simulink model "KalmanAndOnBoardSensors"  (R2015a)
settings: Solver=ode45  StartTime=0.0  StopTime=10.0  RelTol=1e-3
undefined symbols (not defined in the file or in its folder): g, tc
settings Model: Creator=Mattia  LastModifiedBy=Mattia

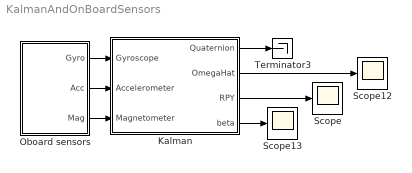
== system KalmanAndOnBoardSensors ==
  Kalman : Subsystem
  Oboard sensors : Subsystem
  Scope : Scope
      settings: SaveName=ScopeData8
  Scope12 : Scope
      settings: SaveName=ScopeData19
  Scope13 : Scope
      settings: SaveName=ScopeData23
  Terminator3 : Terminator
  wires:
  Kalman/1(Quaternion) -> Terminator3/1
  Kalman/2(OmegaHat) -> Scope12/1
  Kalman/3(RPY) -> Scope/1
  Kalman/4(beta) -> Scope13/1
  Oboard sensors/1(Gyro) -> Kalman/1(Gyroscope)
  Oboard sensors/2(Acc) -> Kalman/2(Accelerometer)
  Oboard sensors/3(Mag) -> Kalman/3("Magnetometer ")

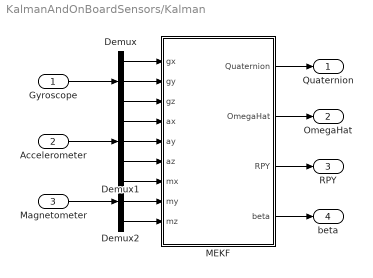
== system KalmanAndOnBoardSensors/Kalman ==
  Gyroscope : Inport
  Accelerometer : Inport  Port=2
  "Magnetometer " : Inport  Port=3
  Demux : Demux  Outputs=3
  Demux1 : Demux  Outputs=3
  Demux2 : Demux  Outputs=3
  MEKF : Subsystem
  Quaternion : Outport
  OmegaHat : Outport  Port=2
  RPY : Outport  Port=3
  beta : Outport  Port=4
  wires:
  Demux1/1 -> MEKF/4(ax)
  Demux1/2 -> MEKF/5(ay)
  Gyroscope/1 -> Demux/1
  Demux1/3 -> MEKF/6(az)
  Demux/3 -> MEKF/3(gz)
  Demux/2 -> MEKF/2(gy)
  Accelerometer/1 -> Demux1/1
  MEKF/2(OmegaHat) -> OmegaHat/1
  MEKF/1(Quaternion) -> Quaternion/1
  MEKF/3(RPY) -> RPY/1
  Demux2/1 -> MEKF/7(mx)
  "Magnetometer "/1 -> Demux2/1
  Demux2/2 -> MEKF/8(my)
  Demux2/3 -> MEKF/9(mz)
  Demux/1 -> MEKF/1(gx)
  MEKF/4("beta ") -> beta/1

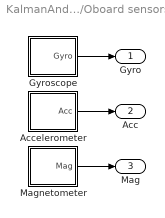
== system KalmanAndOnBoardSensors/Oboard sensors ==
  "Accelerometer " : Subsystem
  "Gyroscope " : Subsystem
  Magnetometer : Subsystem
  Gyro : Outport
  Acc : Outport  Port=2
  Mag : Outport  Port=3
  wires:
  "Gyroscope "/1(Gyro) -> Gyro/1
  "Accelerometer "/1(Acc) -> Acc/1
  Magnetometer/1(Mag) -> Mag/1

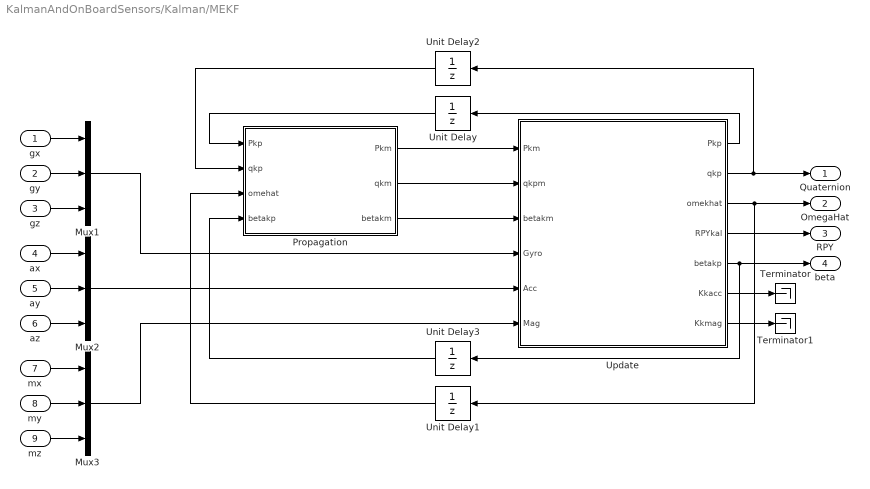
== system KalmanAndOnBoardSensors/Kalman/MEKF ==
  gx : Inport
  gy : Inport  Port=2
  gz : Inport  Port=3
  ax : Inport  Port=4
  ay : Inport  Port=5
  az : Inport  Port=6
  mx : Inport  Port=7
  my : Inport  Port=8
  mz : Inport  Port=9
  Mux1 : Mux  Inputs=3
  Mux2 : Mux  Inputs=3
  Mux3 : Mux  Inputs=3
  "Propagation " : MATLAB Function  TreatAsAtomicUnit=on
  Terminator : Terminator
  Terminator1 : Terminator
  Unit Delay : UnitDelay  InitialCondition=(1e-6)*eye(6)  SampleTime=-1
  Unit Delay1 : UnitDelay  InitialCondition=0.0000001*ones(3,1)  SampleTime=-1
  Unit Delay2 : UnitDelay  InitialCondition=[0 0 0 1]'  SampleTime=-1
  Unit Delay3 : UnitDelay  InitialCondition=0.0000001*ones(3,1)  SampleTime=-1
  Update : MATLAB Function  TreatAsAtomicUnit=on
  Quaternion : Outport
  OmegaHat : Outport  Port=2
  RPY : Outport  Port=3
  "beta " : Outport  Port=4
  wires:
  Update/1(Pkp) -> Unit Delay/1
  Update/3(omekhat) -> Unit Delay1/1, OmegaHat/1
  Unit Delay1/1 -> "Propagation "/3(omehat)
  Unit Delay/1 -> "Propagation "/1(Pkp)
  "Propagation "/1(Pkm) -> Update/1(Pkm)
  gx/1 -> Mux1/1
  gy/1 -> Mux1/2
  ax/1 -> Mux2/1
  mx/1 -> Mux3/1
  az/1 -> Mux2/3
  Update/2(qkp) -> Quaternion/1, Unit Delay2/1
  Update/5(betakp) -> Unit Delay3/1, "beta "/1
  gz/1 -> Mux1/3
  ay/1 -> Mux2/2
  Unit Delay2/1 -> "Propagation "/2(qkp)
  "Propagation "/2(qkm) -> Update/2(qkpm)
  mz/1 -> Mux3/3
  my/1 -> Mux3/2
  Mux1/1 -> Update/4(Gyro)
  Mux2/1 -> Update/5(Acc)
  Mux3/1 -> Update/6(Mag)
  Unit Delay3/1 -> "Propagation "/4(betakp)
  Update/4(RPYkal) -> RPY/1
  "Propagation "/3(betakm) -> Update/3(betakm)
  Update/6(Kkacc) -> Terminator/1
  Update/7(Kkmag) -> Terminator1/1

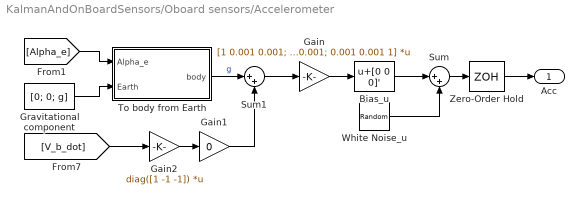
== system KalmanAndOnBoardSensors/Oboard sensors/Accelerometer  ==
  Bias_u : Bias  Bias=[0 0 0]'
  Gain : Gain  Gain=[1 0.001 0.001; 0.001 1 0.001; 0.001 0.001 1]  Multiplication=Matrix(K*u)
  Gain1 : Gain  Gain=0
  Gain2 : Gain  Gain=diag([1 -1 -1])  Multiplication=Matrix(K*u)
  Gravitational component : Constant  Value=[0; 0; g]
  Sum : Sum  Inputs=|++
  Sum1 : Sum  Inputs=|++
  To body from Earth : MATLAB Function  TreatAsAtomicUnit=on
  White Noise_u : RandomNumber  DisableCoverage=on  Variance=0*(0.02)^2  SampleTime=tc
  Zero-Order Hold : ZeroOrderHold  SampleTime=tc
  Acc : Outport
  wires:
  Gain/1 -> Bias_u/1
  Sum1/1 -> Gain/1
  Sum/1 -> Zero-Order Hold/1
  White Noise_u/1 -> Sum/2
  Zero-Order Hold/1 -> Acc/1
  Bias_u/1 -> Sum/1
  Gravitational component/1 -> To body from Earth/2(Earth)
  [Alpha_e] -> To body from Earth/1(Alpha_e)
  To body from Earth/1(body) -> Sum1/1  "g"
  Gain1/1 -> Sum1/2
  [V_b_dot] -> Gain2/1
  Gain2/1 -> Gain1/1

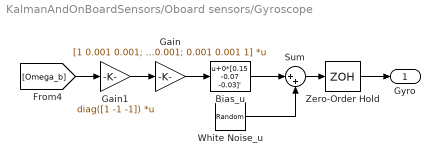
== system KalmanAndOnBoardSensors/Oboard sensors/Gyroscope  ==
  Bias_u : Bias  Bias=0*[0.15 -0.07 -0.03]'
  Gain : Gain  Gain=[1 0.001 0.001; 0.001 1 0.001; 0.001 0.001 1]  Multiplication=Matrix(K*u)
  Gain1 : Gain  Gain=diag([1 -1 -1])  Multiplication=Matrix(K*u)
  Sum : Sum  Inputs=|++
  White Noise_u : RandomNumber  DisableCoverage=on  Variance=0*(0.02)^2  SampleTime=tc
  Zero-Order Hold : ZeroOrderHold  SampleTime=tc
  Gyro : Outport
  wires:
  Bias_u/1 -> Sum/1
  Zero-Order Hold/1 -> Gyro/1
  White Noise_u/1 -> Sum/2
  Sum/1 -> Zero-Order Hold/1
  [Omega_b] -> Gain1/1
  Gain/1 -> Bias_u/1
  Gain1/1 -> Gain/1

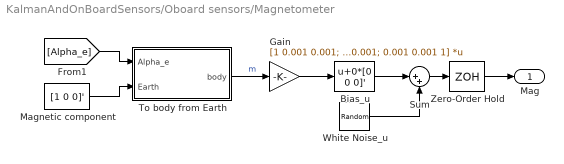
== system KalmanAndOnBoardSensors/Oboard sensors/Magnetometer ==
  Bias_u : Bias  Bias=0*[0 0 0]'
  Gain : Gain  Gain=[1 0.001 0.001; 0.001 1 0.001; 0.001 0.001 1]  Multiplication=Matrix(K*u)
  Magnetic component : Constant  Value=[1 0 0]'
  Sum : Sum  Inputs=|++
  To body from Earth : MATLAB Function  TreatAsAtomicUnit=on
  White Noise_u : RandomNumber  DisableCoverage=on  Variance=0*(0.02)^2  SampleTime=tc
  Zero-Order Hold : ZeroOrderHold  SampleTime=tc
  Mag : Outport
  wires:
  To body from Earth/1(body) -> Gain/1  "m"
  [Alpha_e] -> To body from Earth/1(Alpha_e)
  Magnetic component/1 -> To body from Earth/2(Earth)
  Bias_u/1 -> Sum/1
  Zero-Order Hold/1 -> Mag/1
  White Noise_u/1 -> Sum/2
  Sum/1 -> Zero-Order Hold/1
  Gain/1 -> Bias_u/1

== matlab function KalmanAndOnBoardSensors/Oboard sensors/Accelerometer /To body from Earth ==
  data: Alpha_e input; Earth input; body output
 function body = Tbe(Alpha_e, Earth)
%#codegen
phi = Alpha_e(1);
theta = Alpha_e(2);
psi = Alpha_e(3);

Sphi = sin(phi);
Cphi = cos(phi);
Stheta = sin(theta);
Ctheta = cos(theta);
Spsi = sin(psi);
Cpsi = cos(psi);

TBE = [        Ctheta*Cpsi               Ctheta*Spsi          -Stheta    ;
       Sphi*Stheta*Cpsi-Cphi*Spsi Sphi*Stheta*Spsi+Cphi*Cpsi Sphi*Ctheta ;
       Cphi*Stheta*Cpsi+Sphi*Spsi Cphi*Stheta*Spsi-Sphi*Cpsi Cphi*Ctheta];

body = TBE* Earth;

== matlab function KalmanAndOnBoardSensors/Oboard sensors/Magnetometer/To body from Earth ==
  data: Alpha_e input; Earth input; body output
 function body = Tbe(Alpha_e, Earth)
%#codegen
phi = Alpha_e(1);
theta = Alpha_e(2);
psi = Alpha_e(3);

Sphi = sin(phi);
Cphi = cos(phi);
Stheta = sin(theta);
Ctheta = cos(theta);
Spsi = sin(psi);
Cpsi = cos(psi);

TBE = [        Ctheta*Cpsi               Ctheta*Spsi          -Stheta    ;
       Sphi*Stheta*Cpsi-Cphi*Spsi Sphi*Stheta*Spsi+Cphi*Cpsi Sphi*Ctheta ;
       Cphi*Stheta*Cpsi+Sphi*Spsi Cphi*Stheta*Spsi-Sphi*Cpsi Cphi*Ctheta];

body = TBE* Earth;

== matlab function KalmanAndOnBoardSensors/Kalman/MEKF/Propagation  ==
  data Pkp settings: description=Control signal at the previous step.
  data qkp settings: description=Covariance estimate at the previous step.
  data Pkm settings: description=A-priori covariance estimate.
  data qkm settings: description=A-priori state estimate.
  data: Pkp input; qkp input; Pkm output; qkm output; omehat input; betakp input; betakm output
%% EKF - Propagation      %
% Author: Mattia Giurato  %
% Last review: 2016/03/15 %
%%%%%%%%%%%%%%%%%%%%%%%%%%%
function [Pkm,qkm,betakm] = Propagation(Pkp,qkp,omehat,betakp)
%% Usefull values
sigma_u = diag([0.13807 0.11053 0.063833/10])/100;
sigma_v = diag([0.00001 0.00001 0.05]);
dt = 0.01;

%% Quaternion propagation
omex = [     0      -omehat(3)  omehat(2) ;
         omehat(3)      0      -omehat(1) ;
        -omehat(2)  omehat(1)      0     ];
Omega = [  -omex   omehat ;
         -omehat'     0  ];
qt = (eye(4) + .5*Omega*dt)*qkp;
qkm = qt / sqrt(qt(1)^2+qt(2)^2+qt(3)^2+qt(4)^2);

%% Bias propagation
betakm = betakp;

%% Covariance equation propagation
omekhatx = [     0      -omehat(3)  omehat(2) ;
             omehat(3)     0       -omehat(1) ;
            -omehat(2)  omehat(1)      0     ];
nomehat = sqrt(omehat(1)^2+omehat(2)^2+omehat(3)^2);
Phi1 = eye(3) - omekhatx*sin(nomehat*dt)/nomehat + omekhatx*omekhatx*(1 - cos(nomehat*dt))/(nomehat^2);
Phi2 = omekhatx*(1 - cos(nomehat*dt))/(nomehat^2) - eye(3)*dt - omekhatx*omekhatx*(nomehat*dt - sin(nomehat*dt))/(nomehat^3);
Phi = [  Phi1    Phi2  ;
       zeros(3) eye(3)];
gamma = [-eye(3) zeros(3) ;
         zeros(3) eye(3) ];
Q = [(sigma_v^2*dt + 1/3*sigma_u^2*dt^3)*eye(3) (.5*sigma_u^2*dt^2)*eye(3) ;
             (.5*sigma_u^2*dt^2)*eye(3)            (sigma_u^2*dt)*eye(3)  ];
Pkm = Phi*Pkp*Phi' + gamma*Q*gamma';

== matlab function KalmanAndOnBoardSensors/Kalman/MEKF/Update ==
  data Pkm settings: description=A-priori state estimate.
  data qkpm settings: description=A-priori covariance estimate.
  data betakm settings: description=Measurements from the sensors.
  data Pkp settings: description=Corrected state estimate.
  data omekhat settings: description=Corrected covariance estimate.
  data: Pkm input; qkpm input; betakm input; Gyro input; Pkp output; qkp output; omekhat output; RPYkal output; Acc input; Mag input; betakp output; Kkacc output; Kkmag output
%% EKF - Update           %
% Author: Mattia Giurato  %
% Last review: 2016/03/15 %
%%%%%%%%%%%%%%%%%%%%%%%%%%%
function [Pkp,qkp,omekhat,RPYkal,betakp,Kkacc,Kkmag] = Update(Pkm,qkpm,betakm,Gyro,Acc,Mag)
gx = Gyro(1);
gy = Gyro(2);
gz = Gyro(3);
ax = Acc(1);
ay = Acc(2);
az = Acc(3);
mx = Mag(1);
my = Mag(2);
mz = Mag(3);
Gyroscope = [gx gy gz]';
Accelerometer = [ax ay az]';
Magnetometer = [mx my mz]';

% Usefull values
sigma_acc = diag([0.77418 0.66936 0.71485]);
sigma_mag = 300*diag([0.053667 0.034382 0.071054]);

% Normalise accelerometer measurement
% if(norm(Accelerometer) == 0), return; end % handle NaN
b_acc = Accelerometer / sqrt(ax^2 + ay^2 + az^2); % normalise magnitude

% Normalise magnetometer measurement
% if(norm(Magnetometer) == 0), return; end % handle NaN
b_mag = Magnetometer / sqrt(mx^2 + my^2 + mz^2); % normalise magnitude

%% Propagated value from previous step
deltaXkm = zeros(6,1);

  %% Accelerometer and Magnetometer correction     
  % Compute attitude matrix
  ro = [qkpm(1) ;
        qkpm(2) ;
        qkpm(3)];
  q_4 = qkpm(4);
  rox = [   0   -ro(3)  ro(2) ;
           ro(3)  0    -ro(1) ;
          -ro(2) ro(1)   0   ];
  normrosq = ro(1)^2+ro(2)^2+ro(3)^2;
  Aqkpm = (q_4^2 - normrosq)*eye(3) + 2*(ro*ro') - 2*q_4*rox;
  
  % Reference direction of Earth's gravitational field
  r_acc = [0 ;
           0 ;
           1];
  Aqmr = Aqkpm*r_acc;
  b = b_acc;
  R = sigma_acc^2*eye(3);
  
  % Sensitivity Matrix
  Aqmrx = [      0   -Aqmr(3)  Aqmr(2) ;
             Aqmr(3)    0     -Aqmr(1) ;
            -Aqmr(2)  Aqmr(1)    0    ];
  Hk = [Aqmrx zeros(3)];
  
  % Gain
  Kkacc = (Pkm*Hk')/(Hk*Pkm*Hk' + R);
  
  % Update Covariance
  Pkp = (eye(6) - Kkacc*Hk)*Pkm*(eye(6) - Kkacc*Hk)' + Kkacc*R*Kkacc';
  
  % Update state
  epk = b - Aqmr; %residual
  yk = epk - Hk*deltaXkm;
  deltaXkp = diag([1 1 0 1 1 0])*Kkacc*yk;
  
  % Update quaternion
  dalphak = deltaXkp(1:3,1);
  dq = (1/sqrt(4+(dalphak(1)^2+dalphak(2)^2+dalphak(3)^2)))*[dalphak' 2]';
  qkp = [dq(4)*ro + q_4*dq(1:3,1)-cross(dq(1:3,1),ro) ;
                 dq(4)*q_4 - dot(dq(1:3,1),ro)       ];
  
  % Update biases
  deltaBeta = deltaXkp(4:6,1);
  betakp = betakm + deltaBeta;
  
  Pkm = Pkp;
  deltaXkm = deltaXkp;
  betakm = betakp;
  qkpm = qkp;
  
  % Compute attitude matrix
  ro = [qkpm(1) ;
        qkpm(2) ;
        qkpm(3)];
  q_4 = qkpm(4);
  rox = [   0   -ro(3)  ro(2) ;
           ro(3)  0    -ro(1) ;
          -ro(2) ro(1)   0   ];
  normrosq = ro(1)^2+ro(2)^2+ro(3)^2;
  Aqkpm = (q_4^2 - normrosq)*eye(3) + 2*(ro*ro') - 2*q_4*rox;
  
  % Reference direction of Earth's magnetic feild
  h = Aqkpm*Magnetometer;
  r_mag = [sqrt(h(1)^2 + h(2)^2) ;
                      0          ;
                     h(3)       ];
  Aqmr = Aqkpm*r_mag;
  b = b_mag;
  R = sigma_mag^2*eye(3);
  
  % Sensitivity Matrix
  Aqmrx = [      0   -Aqmr(3)  Aqmr(2) ;
             Aqmr(3)    0     -Aqmr(1) ;
            -Aqmr(2)  Aqmr(1)    0    ];
  Hk = [Aqmrx zeros(3)];
  
  % Gain
  Kkmag = (Pkm*Hk')/(Hk*Pkm*Hk' + R);
  
  % Update Covariance
  Pkp = (eye(6) - Kkmag*Hk)*Pkm*(eye(6) - Kkmag*Hk)' + Kkmag*R*Kkmag';
  
  % Update state
  epk = b - Aqmr; %residual
  yk = epk - Hk*deltaXkm;
  deltaXkp = diag([0 0 1 0 0 1])*(deltaXkm + Kkmag*yk);
  
  % Update quaternion
  dalphak = deltaXkp(1:3,1);
  dq = (1/sqrt(4+(dalphak(1)^2+dalphak(2)^2+dalphak(3)^2)))*[dalphak' 2]';
  qkp = [dq(4)*ro + q_4*dq(1:3,1)-cross(dq(1:3,1),ro) ;
                 dq(4)*q_4 - dot(dq(1:3,1),ro)       ];
  
  % Update biases
  deltaBeta = deltaXkp(4:6,1);
  betakp = betakm + deltaBeta;
  
%% Depolarize gyroscope measurement
omekhat = Gyroscope - betakp;

%% Convert Quaternion into RPY
a1 = 2.*(qkp(1).*qkp(2) + qkp(4).*qkp(3));
a2 = qkp(4).^2 + qkp(1).^2 - qkp(2).^2 - qkp(3).^2;
b = -2.*(qkp(1).*qkp(3) - qkp(4).*qkp(2));
c1 = 2.*(qkp(2).*qkp(3) + qkp(4).*qkp(1));
c2 = qkp(4).^2 - qkp(1).^2 - qkp(2).^2 + qkp(3).^2;

Yy = atan2( a1, a2 );
Pp = asin( b );
Rr = atan2( c1, c2 );

RPYkal = [Rr -Pp -Yy]';
